simulink model "sim_switc_hover_vol_rotation"  (R2020b)
settings: Solver=VariableStepAuto  StartTime=0.0  StopTime=T  MaxStep=MaxStep  RelTol=RelTol
values from neighbouring files (symbols this model uses):
  a = 400    [switch_hovering_vol_rotation.m]
  b = 500    [switch_hovering_vol_rotation.m]
  controlleur = generateContolleur(drone)    [switch_hovering_vol_rotation.m]
  drone = generateDarko()    [switch_hovering_vol_rotation.m]
  J = 200    [switch_hovering_vol_rotation.m]
  K_complet = [K(:,1:6), [0;0;0;0], K(:,7:12)]    [switch_hovering_vol_rotation.m]
  rule = 1    [switch_hovering_vol_rotation.m]
  S_complet = [S(1:6,1:6), zeros(6,1), S(1:6,7:12); zeros(1,13); S(7:12,1:6), zeros(6,1), S(7:12,7:12)]    [switch_hovering_vol_rotation.m]
  T = 80    [switch_hovering_vol_rotation.m]
  u_eq_hover = drone.G*drone.MASS/(2*drone.Fb(1,1)) * [1;1;0;0]    [switch_hovering_vol_rotation.m]
  x0 = [p_initial; v_initial; q_initial; omega_initial; s]    [switch_hovering_vol_rotation.m]
  x_eq_hover = [[0; 0; 0]; [0; 0; 0]; [1/sqrt(2); 0; -1/sqrt(2);0]; [0; 0; 0]]    [switch_hovering_vol_rotation.m]
undefined symbols (not defined in the file or in its folder): f_initial, q_d_initial, speed
libraries: simulink_extras x5, simulink x3, pid_lib x1, sharedtransform x1
(part 1 of 2)
settings Model: Creator=florian  LastModifiedBy=florian

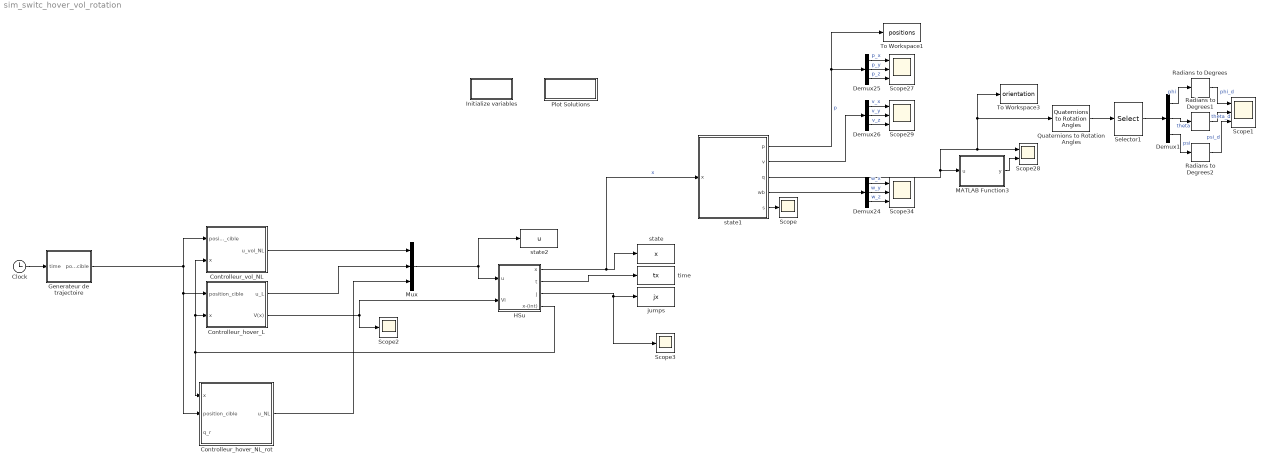
== system sim_switc_hover_vol_rotation ==
  Clock : Clock
  Controlleur_hover_L : Subsystem
  Controlleur_hover_NL_rot : Subsystem
  Controlleur_vol_NL : Subsystem
  Demux{1,24..26} (4 alike) : Demux  Outputs=3
  Generateur de trajectoire : MATLAB Function  TreatAsAtomicUnit=on
  HSu : Subsystem  LoadFcn=set_param(gcb,'LinkStatus','none')
      settings: CopyFcn=|
      | set_param(gcb,'LinkStatus','none'),
      | set_param(gcs, 'MaxStep', 'MaxStep', 'RelTol', 'RelTol','Stop time', 'T')
      mask Display:
      | image(imread('Hcal.jpg'))
      | %plot([5 20 20 5 5],[5 5 20 20 5])
      | %text(8,13,'HyEq_mdl')
      | port_label('output', 1, 'x')
      | port_label('output', 2, 't')
      | port_label('output', 3, 'j')
      | port_label('output', 4, 'x-(int)')
      | port_label('input', 1, 'u')
      | port_label('input', 2, 'V(x)')
  Initialize variables : Subsystem  Priority=-10
      settings: OpenFcn=initialization_di
      mask Display: disp('Double Click\n to Initialize')
  MATLAB Function3 : MATLAB Function  TreatAsAtomicUnit=on
  Mux : Mux  Inputs=3
  Plot Solutions : Subsystem
      settings: OpenFcn=postprocessing_di
      mask Display: disp('Double Click to\n Plot Solutions')
  Quaternions to Rotation Angles : sharedtransform/Quaternions to Rotation Angles  rotationOrder=ZXY  aMode=aMode
      settings: SourceProductBaseCode=AE,PW,MT,UV,VE,VP
  Radians to Degrees : simulink_extras/Transformations/Radians to Degrees
  Radians to Degrees1 : simulink_extras/Transformations/Radians to Degrees
  Radians to Degrees2 : simulink_extras/Transformations/Radians to Degrees
  Scope : Scope
  Scope{1,27,29,34} (4 alike) : Scope  NumInputPorts=3
  Scope2 : Scope
  Scope28 : Scope  NumInputPorts=2
  Scope3 : Scope
  Selector1 : Selector  InputPortWidth=3  IndexOptions=Index vector (dialog)  Indices=[2 3 1]  OutputSizes=1
  To Workspace1 : ToWorkspace  VariableName=positions  SampleTime=-1
  To Workspace3 : ToWorkspace  VariableName=orientation  SampleTime=-1
  jumps : ToWorkspace  VariableName=jx  SampleTime=-1
  state : ToWorkspace  VariableName=x  SampleTime=-1
  state1 : MATLAB Function  TreatAsAtomicUnit=on
  state2 : ToWorkspace  VariableName=u  SampleTime=-1
  time : ToWorkspace  VariableName=tx  SampleTime=-1
  wires:
  Mux/1 -> HSu/1(u), state2/1
  HSu/1(x) -> state1/1(x), state/1  "x"
  HSu/2(t) -> time/1
  HSu/3(j) -> jumps/1, Scope3/1
  Controlleur_hover_L/1(u_L) -> Mux/2
  Generateur de trajectoire/1(position_cible) -> Controlleur_vol_NL/1(position_cible), Controlleur_hover_NL_rot/2(position_cible), Controlleur_hover_L/1(position_cible)
  Controlleur_hover_L/2(V(x)) -> Scope2/1, HSu/2(Vi)
  HSu/4(x-(int)) -> Controlleur_hover_NL_rot/1(x), Controlleur_vol_NL/2(x), Controlleur_hover_L/2(x)
  Demux1/2 -> Radians to Degrees1/1  "theta"
  Quaternions to Rotation Angles/1 -> Selector1/1
  Demux1/3 -> Radians to Degrees2/1  "psi"
  Demux24/2 -> Scope34/2  "w_y"
  Demux26/3 -> Scope29/3  "v_z"
  state1/1(p) -> To Workspace1/1, Demux25/1  "p"
  Demux25/3 -> Scope27/3  "p_z"
  Demux1/1 -> Radians to Degrees/1  "phi"
  Demux25/1 -> Scope27/1  "p_x"
  state1/3(q) -> Scope28/1, To Workspace3/1, Quaternions to Rotation Angles/1, MATLAB Function3/1(u)
  Selector1/1 -> Demux1/1
  Radians to Degrees/1 -> Scope1/1  "phi_d"
  Radians to Degrees1/1 -> Scope1/2  "theta_d"
  Radians to Degrees2/1 -> Scope1/3  "psi_d"
  MATLAB Function3/1(y) -> Scope28/2
  state1/2(v) -> Demux26/1
  Demux26/2 -> Scope29/2  "v_y"
  Demux24/3 -> Scope34/3  "w_z"
  state1/4(wb) -> Demux24/1
  Demux24/1 -> Scope34/1  "w_x"
  Demux26/1 -> Scope29/1  "v_x"
  Demux25/2 -> Scope27/2  "p_y"
  state1/5(s) -> Scope/1
  Controlleur_vol_NL/1(u_vol_NL) -> Mux/1
  Controlleur_hover_NL_rot/1(u_NL) -> Mux/3
  Clock/1 -> Generateur de trajectoire/1(time)

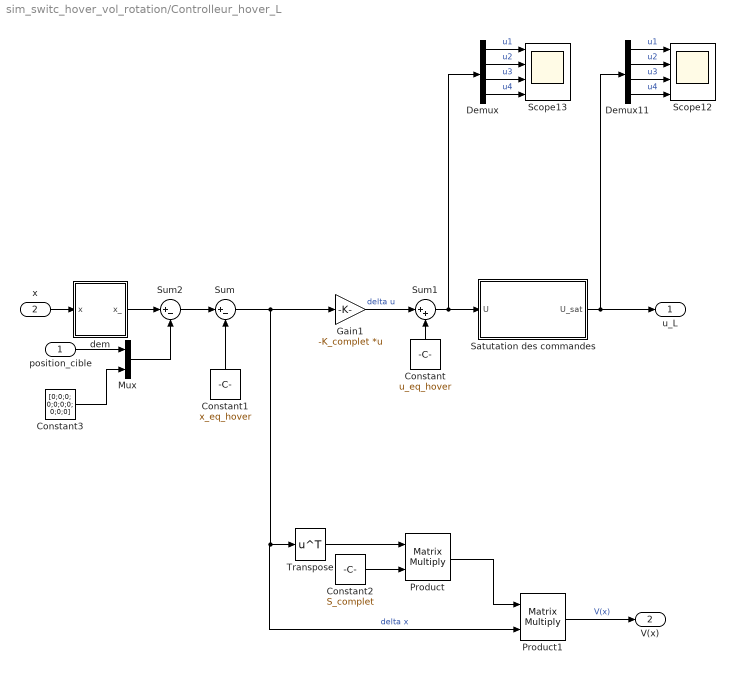
== system sim_switc_hover_vol_rotation/Controlleur_hover_L ==
  position_cible : Inport
  x : Inport  Port=2
  Constant : Constant  Value=u_eq_hover
  Constant1 : Constant  Value=x_eq_hover
  Constant2 : Constant  Value=S_complet
  Constant3 : Constant  Value=[0;0;0; 0;0;0;0; 0;0;0]
  Demux : Demux
  Demux11 : Demux
  Gain1 : Gain  Gain=-K_complet  Multiplication=Matrix(K*u) (u vector)
  Mux : Mux  Inputs=2
  Product : Product  Multiplication=Matrix(*)
  Product1 : Product  Multiplication=Matrix(*)
  Satutation des commandes : Subsystem
  Scope12 : Scope  NumInputPorts=4
  Scope13 : Scope  NumInputPorts=4
  Sum : Sum  Inputs=|+-
  Sum1 : Sum  Inputs=|++
  Sum2 : Sum  Inputs=|+-
  Transpose : Math  Operator=transpose  SaturateOnIntegerOverflow=on
  dem : MATLAB Function  TreatAsAtomicUnit=on
  u_L : Outport
  V(x) : Outport  Port=2
  wires:
  Demux/1 -> Scope13/1  "u1"
  Demux/3 -> Scope13/3  "u3"
  Gain1/1 -> Sum1/1  "delta u"
  Sum1/1 -> Satutation des commandes/1(U), Demux/1
  Sum/1 -> Gain1/1, Product1/2, Transpose/1  "delta x"
  Demux11/3 -> Scope12/3  "u3"
  Satutation des commandes/1(U_sat) -> u_L/1, Demux11/1
  Demux11/2 -> Scope12/2  "u2"
  Product1/1 -> V(x)/1  "V(x)"
  Demux/4 -> Scope13/4  "u4"
  Constant1/1 -> Sum/2
  Transpose/1 -> Product/1
  Product/1 -> Product1/1
  Constant/1 -> Sum1/2
  Demux11/4 -> Scope12/4  "u4"
  Demux/2 -> Scope13/2  "u2"
  Constant2/1 -> Product/2
  Sum2/1 -> Sum/1
  Demux11/1 -> Scope12/1  "u1"
  Mux/1 -> Sum2/2
  position_cible/1 -> Mux/1
  Constant3/1 -> Mux/2
  x/1 -> dem/1(x)
  dem/1(x_) -> Sum2/1

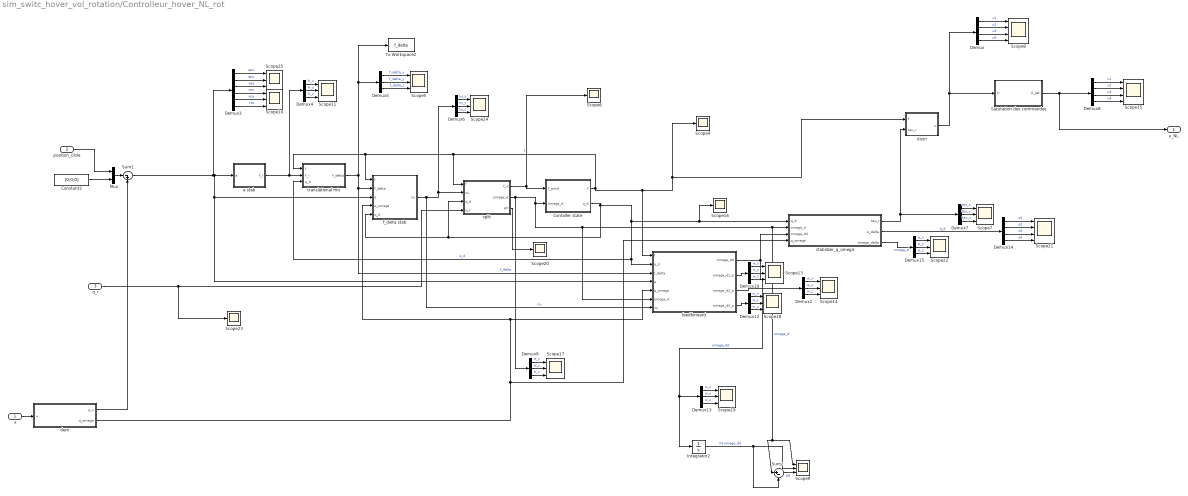
== system sim_switc_hover_vol_rotation/Controlleur_hover_NL_rot ==
  x : Inport
  position_cible : Inport  Port=2
  q_r : Inport  Port=3
  Constant2 : Constant  Value=[0;0;0]
  Contoller state : Subsystem
  Demux : Demux
  Demux{2,4..7,9..10,12..13,15} (10 alike) : Demux  Outputs=3
  Demux14 : Demux
  Demux3 : Demux  Outputs=6
  Demux8 : Demux
  Integrator2 : Integrator
  Mux : Mux  Inputs=2
  Satutation des commandes : Subsystem
  Scope{5,7,9..11,13..14,17..19,22,24..25} (13 alike) : Scope  NumInputPorts=3
  Scope15 : Scope  NumInputPorts=4
  Scope{4,6,16,20,23} (5 alike) : Scope
  Scope21 : Scope  NumInputPorts=4
  Scope8 : Scope  NumInputPorts=4
  Sum1 : Sum  Inputs=|-+
  Sum2 : Sum  Inputs=|+-
  To Workspace2 : ToWorkspace  VariableName=f_delta  SampleTime=-1
  dem : MATLAB Function  TreatAsAtomicUnit=on
  distri : MATLAB Function  TreatAsAtomicUnit=on
  e stab : MATLAB Function  TreatAsAtomicUnit=on
  f_delta stab : MATLAB Function  TreatAsAtomicUnit=on
  feedforward : MATLAB Function  TreatAsAtomicUnit=on
  split : MATLAB Function  TreatAsAtomicUnit=on
  stabilizer_q_omega : MATLAB Function  TreatAsAtomicUnit=on
  translational mis : MATLAB Function  TreatAsAtomicUnit=on
  u_NL : Outport
  wires:
  Demux3/3 -> Scope25/3  "epz"
  Demux15/2 -> Scope22/2  "w_y"
  feedforward/1(omega_dd) -> stabilizer_q_omega/3(omega_dd), Demux13/1, Integrator2/1  "omega_dd"
  split/2(omega_d) -> Demux9/1, feedforward/6(omega_d), Sum2/1, Scope9/1, stabilizer_q_omega/2(omega_d), Contoller state/2(omega_d)  "omega_d"
  Demux3/2 -> Scope25/2  "epy"
  Demux8/4 -> Scope15/4  "u4"
  Demux6/1 -> Scope24/1  "nu_x"
  translational mis/1(f_delta) -> Demux5/1, To Workspace2/1, feedforward/3(f_delta), f_delta stab/2(f_delta)  "f_delta"
  Demux7/2 -> Scope7/2  "tau_y"
  feedforward/3(omega_d2_p) -> Demux2/1
  Demux3/1 -> Scope25/1  "epx"
  Demux8/3 -> Scope15/3  "u3"
  Constant2/1 -> Mux/2
  Demux7/3 -> Scope7/3  "tau_z"
  Demux/3 -> Scope8/3  "u3"
  Demux10/1 -> Scope13/1  "w_x"
  position_cible/1 -> Mux/1
  Demux7/1 -> Scope7/1  "tau_x"
  Satutation des commandes/1(U_sat) -> u_NL/1, Demux8/1
  Demux13/2 -> Scope19/2  "w_y"
  Sum1/1 -> Demux3/1, feedforward/4(e), f_delta stab/3(e), e stab/1(e)
  Demux4/1 -> Scope11/1  "fr_x"
  Demux5/3 -> Scope5/3  "f_delta_z"
  Demux14/1 -> Scope21/1  "q1"
  e stab/1(f_r) -> Demux4/1, translational mis/2(f_r)
  f_delta stab/1(nu) -> feedforward/7(nu), Demux6/1, split/2(nu)  "nu"
  Demux12/2 -> Scope18/2  "w_y"
  q_r/1 -> split/4(q_r), Scope23/1
  Demux6/3 -> Scope24/3  "nu_z"
  Demux8/1 -> Scope15/1  "u1"
  Demux10/2 -> Scope13/2  "w_y"
  Demux9/1 -> Scope17/1  "w_x"
  Mux/1 -> Sum1/1
  Demux12/1 -> Scope18/1  "w_x"
  feedforward/4(omega_d3_p) -> Demux12/1
  Demux/4 -> Scope8/4  "u4"
  Demux8/2 -> Scope15/2  "u2"
  Demux15/1 -> Scope22/1  "w_x"
  Demux5/2 -> Scope5/2  "f_delta_y"
  Demux10/3 -> Scope13/3  "w_z"
  Integrator2/1 -> Sum2/2, Scope9/2  "int omega_dd"
  Demux15/3 -> Scope22/3  "w_z"
  Demux9/2 -> Scope17/2  "w_y"
  Demux2/2 -> Scope14/2  "w_y"
  Demux2/3 -> Scope14/3  "w_z"
  dem/2(q_omega) -> stabilizer_q_omega/4(q_omega), feedforward/5(q_omega), f_delta stab/4(q_omega)
  Demux12/3 -> Scope18/3  "w_z"
  Contoller state/1(f) -> f_delta stab/1(f), translational mis/1(f), split/1(f), feedforward/1(f), Scope4/1, distri/1(f)  "f"
  Demux6/2 -> Scope24/2  "nu_y"
  split/1(f_d) -> Scope6/1, Contoller state/1(f_point)
  Demux/2 -> Scope8/2  "u2"
  Demux13/3 -> Scope19/3  "w_z"
  Demux9/3 -> Scope17/3  "w_z"
  Demux3/4 -> Scope10/1  "vpx"
  Demux2/1 -> Scope14/1  "w_x"
  Demux4/3 -> Scope11/3  "fr_z"
  Contoller state/2(q_d) -> f_delta stab/5(q_d), split/3(q_d), feedforward/2(q_d), translational mis/3(q_d), Scope16/1, stabilizer_q_omega/1(q_d)  "q_d"
  Demux13/1 -> Scope19/1  "w_x"
  Demux3/5 -> Scope10/2  "vpy"
  Demux5/1 -> Scope5/1  "f_delta_x"
  Demux3/6 -> Scope10/3  "vpz"
  Sum2/1 -> Scope9/3  "dif"
  Demux14/2 -> Scope21/2  "q2"
  dem/1(p_v) -> Sum1/2
  Demux4/2 -> Scope11/2  "fr_y"
  stabilizer_q_omega/2(q_delta) -> Demux14/1  "q_d"
  split/3(err) -> Scope20/1
  Demux14/4 -> Scope21/4  "q4"
  Demux/1 -> Scope8/1  "u1"
  stabilizer_q_omega/1(tau_r) -> distri/2(tau_r), Demux7/1
  feedforward/2(omega_d1_p) -> Demux10/1
  stabilizer_q_omega/3(omega_delta) -> Demux15/1  "omega_d"
  distri/1(u) -> Satutation des commandes/1(U), Demux/1
  Demux14/3 -> Scope21/3  "q3"
  x/1 -> dem/1(x)

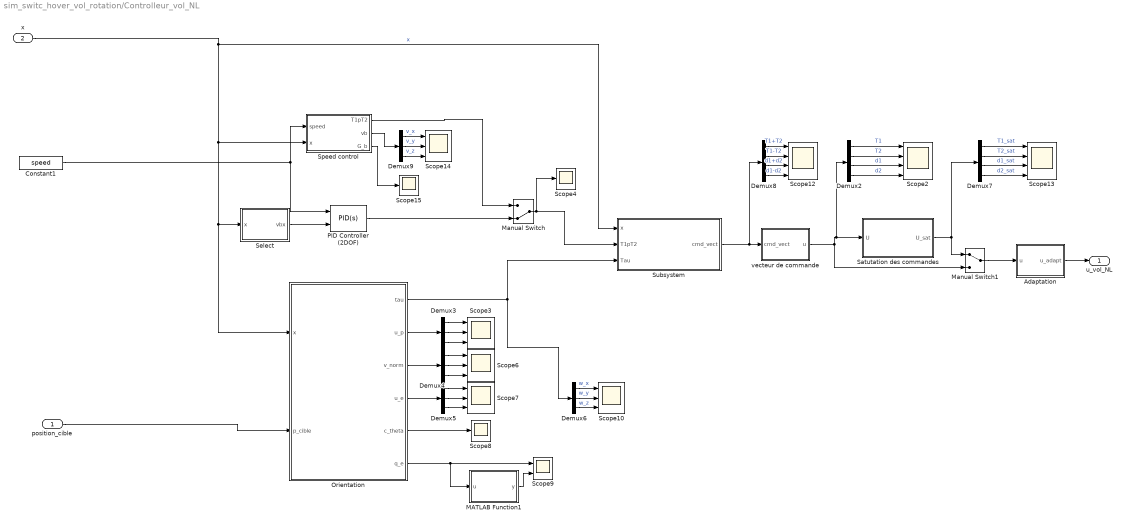
== system sim_switc_hover_vol_rotation/Controlleur_vol_NL ==
  position_cible : Inport
  x : Inport  Port=2
  Adaptation : MATLAB Function  TreatAsAtomicUnit=on
  Constant1 : Constant  Value=speed
  Demux2 : Demux
  Demux{3..6,9} (5 alike) : Demux  Outputs=3
  Demux7 : Demux
  Demux8 : Demux
  MATLAB Function1 : MATLAB Function  TreatAsAtomicUnit=on
  Manual Switch : ManualSwitch  CurrentSetting=0
  Manual Switch1 : ManualSwitch
  Orientation : MATLAB Function  TreatAsAtomicUnit=on
  PID Controller (2DOF) : pid_lib/PID Controller (2DOF)  Controller=PID  Form=Parallel  TimeDomain=Continuous-time  UseExternalTs=off  SampleTime=-1  IntegratorMethod=Forward Euler  FilterMethod=Forward Euler  ControllerParametersSource=internal  P=1  I=1  D=0.1  UseFilter=on  N=100  b=1  c=1  TunerSelectOption=Transfer Function Based (PID Tuner App)  InitialConditionSource=internal  InitialConditionForIntegrator=0  InitialConditionForFilter=0  DifferentiatorICPrevScaledInput=0  ExternalReset=none  TrackingMode=off  Kt=1  LimitOutput=off  SatLimitsSource=internal  UpperSaturationLimit=inf  LowerSaturationLimit=-inf  LinearizeAsGain=on  AntiWindupMode=none  Kb=1  POutMin=[]  POutMax=[]  IOutMin=[]  IOutMax=[]  DOutMin=[]  DOutMax=[]  NOutMin=[]  NOutMax=[]  bOutMin=[]  bOutMax=[]  cOutMin=[]  cOutMax=[]  SumOutMin=[]  SumOutMax=[]  SaturationOutMin=[]  SaturationOutMax=[]  PParamMin=[]  PParamMax=[]  IParamMin=[]  IParamMax=[]  DParamMin=[]  DParamMax=[]  NParamMin=[]  NParamMax=[]  bParamMin=[]  bParamMax=[]  cParamMin=[]  cParamMax=[]  KbParamMin=[]  KbParamMax=[]  KtParamMin=[]  KtParamMax=[]  KbOutMin=[]  KbOutMax=[]  KtOutMin=[]  KtOutMax=[]  IntegratorOutMin=[]  IntegratorOutMax=[]  FilterOutMin=[]  FilterOutMax=[]  SumI1OutMin=[]  SumI1OutMax=[]  SumI2OutMin=[]  SumI2OutMax=[]  SumI3OutMin=[]  SumI3OutMax=[]  SumI4OutMin=[]  SumI4OutMax=[]  SumDOutMin=[]  SumDOutMax=[]  Sum1OutMin=[]  Sum1OutMax=[]  Sum2OutMin=[]  Sum2OutMax=[]  Sum3OutMin=[]  Sum3OutMax=[]  DifferentiatorOutMin=[]  DifferentiatorOutMax=[]  FilterDiffOutCoefMin=[]  FilterDiffOutCoefMax=[]  ReciprocalOutMin=[]  ReciprocalOutMax=[]  SumDenOutMin=[]  SumDenOutMax=[]  SumNumOutMin=[]  SumNumOutMax=[]  DivideOutMin=[]  DivideOutMax=[]  UdiffTsProdOutMin=[]  UdiffTsProdOutMax=[]  NTsProdOutMin=[]  NTsProdOutMax=[]  UintegralTsProdOutMin=[]  UintegralTsProdOutMax=[]  UngainTsProdOutMin=[]  UngainTsProdOutMax=[]  IntegratorContinuousStateAttributes=''  IntegratorStateMustResolveToSignalObject=off  IntegratorRTWStateStorageClass=Auto  FilterContinuousStateAttributes=''  FilterStateMustResolveToSignalObject=off  FilterRTWStateStorageClass=Auto  ParallelPVariant=InternalParameters  IdealPVariant=Disabled  IVariant=InternalParameters  DVariant=InternalParameters  bVariant=InternalParameters  cVariant=InternalParameters  IntegratorVariant=Continuous  SatVariant=Disabled  AWVariant=Passthrough  PCopyVariant=Disabled  TRVariant=Disabled  FdbkBlocksVariant=Forward  IdealPFdbkVariant=Disabled  SatFdbkVariant=Disabled  DerivativeFilterVariant=ContFilter  NVariant=InternalParameters  NCopyVariant=Disabled  FilterICVariant=InternalICsFilter  IntegratorICVariant=InternalICs  ExternalResetVariant=Disabled  TRSumVariant=Passthrough  SumFdbkVariant=Disabled  SumVariant=Sum_PID  TsampFilterVariant=InternalTs  TsampNgainVariant=Passthrough  TsampIntegralVariant=Passthrough  ExternalSaturationOutDataTypeStr=Inherit: Same as second input
      settings: SourceProductBaseCode=SL
  Satutation des commandes : Subsystem
  Scope{3,6..7,10,14} (5 alike) : Scope  NumInputPorts=3
  Scope12 : Scope  NumInputPorts=4
  Scope13 : Scope  NumInputPorts=4
  Scope15 : Scope
  Scope2 : Scope  NumInputPorts=4
  Scope4 : Scope
  Scope8 : Scope
  Scope9 : Scope  NumInputPorts=2
  Select : MATLAB Function  TreatAsAtomicUnit=on
  Speed control : MATLAB Function  TreatAsAtomicUnit=on
  Subsystem : Subsystem
  vecteur de commande : MATLAB Function  TreatAsAtomicUnit=on
  u_vol_NL : Outport
  wires:
  Orientation/4(u_e) -> Demux5/1
  Demux7/1 -> Scope13/1  "T1_sat"
  Demux5/2 -> Scope7/2
  Demux9/3 -> Scope14/3  "v_z"
  Orientation/5(c_theta) -> Scope8/1
  Subsystem/1(cmd_vect) -> Demux8/1, vecteur de commande/1(cmd_vect)
  Demux2/3 -> Scope2/3  "d1"
  Speed control/2(vb) -> Demux9/1
  Orientation/6(q_e) -> MATLAB Function1/1(u), Scope9/1
  Demux6/2 -> Scope10/2  "w_y"
  x/1 -> Subsystem/1(x), Select/1(x), Orientation/1(x), Speed control/2(x)  "x"
  Orientation/3(v_norm) -> Demux4/1
  Orientation/2(u_p) -> Demux3/1
  Demux6/1 -> Scope10/1  "w_x"
  Select/1(vbx) -> PID Controller (2DOF)/2
  Demux6/3 -> Scope10/3  "w_z"
  MATLAB Function1/1(y) -> Scope9/2
  Demux8/3 -> Scope12/3  "d1+d2"
  Orientation/1(tau) -> Subsystem/3(Tau), Demux6/1
  Demux8/4 -> Scope12/4  "d1-d2"
  Demux2/4 -> Scope2/4  "d2"
  Demux4/1 -> Scope6/1
  Demux9/1 -> Scope14/1  "v_x"
  Demux8/2 -> Scope12/2  "T1-T2"
  Demux4/2 -> Scope6/2
  Demux5/3 -> Scope7/3
  Manual Switch/1 -> Scope4/1, Subsystem/2(T1pT2)
  Demux9/2 -> Scope14/2  "v_y"
  Demux7/2 -> Scope13/2  "T2_sat"
  Satutation des commandes/1(U_sat) -> Demux7/1, Manual Switch1/1
  Demux5/1 -> Scope7/1
  Demux3/1 -> Scope3/1
  Speed control/1(T1pT2) -> Manual Switch/1
  Demux2/1 -> Scope2/1  "T1"
  PID Controller (2DOF)/1 -> Manual Switch/2
  Constant1/1 -> Speed control/1(speed), PID Controller (2DOF)/1
  Demux3/3 -> Scope3/3
  Speed control/3(G_b) -> Scope15/1
  Demux8/1 -> Scope12/1  "T1+T2"
  Demux2/2 -> Scope2/2  "T2"
  Demux4/3 -> Scope6/3
  Demux7/3 -> Scope13/3  "d1_sat"
  Demux7/4 -> Scope13/4  "d2_sat"
  vecteur de commande/1(u) -> Demux2/1, Satutation des commandes/1(U), Manual Switch1/2
  Demux3/2 -> Scope3/2
  Manual Switch1/1 -> Adaptation/1(u)
  Adaptation/1(u_adapt) -> u_vol_NL/1
  position_cible/1 -> Orientation/2(p_cible)

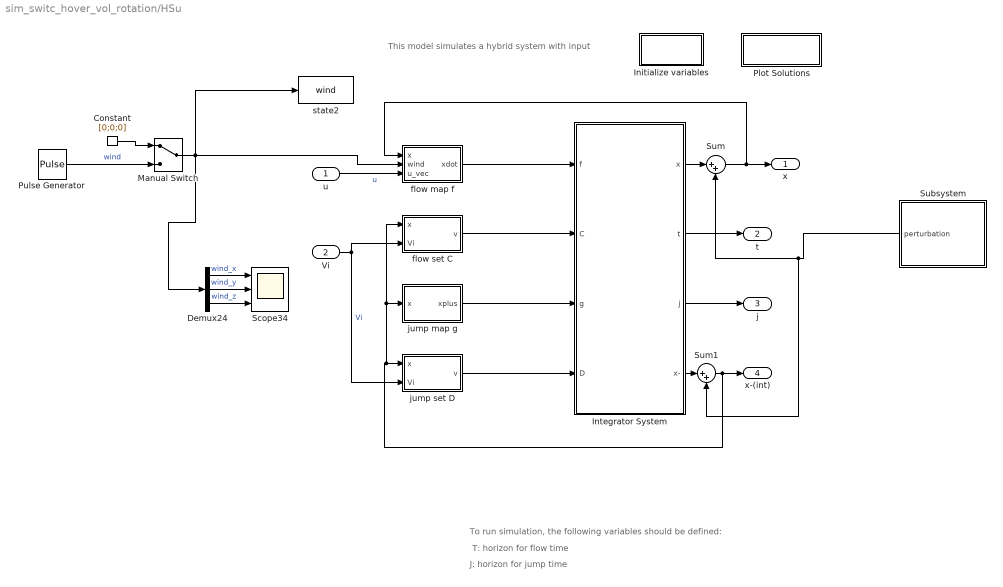
== system sim_switc_hover_vol_rotation/HSu ==
  note: J: horizon for jump time
  note: T: horizon for flow time
  note: To run simulation, the following variables should be defined:
  note: This model simulates a hybrid system with input
  u : Inport
  Vi : Inport  Port=2
  Constant : Constant  Value=[0;0;0]
  Demux24 : Demux  Outputs=3
  Initialize variables : Subsystem  Priority=-10
      settings: OpenFcn=|
      | try
      |      clearvars -except inifile pathfile_in pathfile_pos posfile
      |      cd(pathfile_in);
      |      eval(inifile);
      | catch
      |      [inifile,pathfile_in] = getInitializationfile;
      |      cd(pathfile_in);
      |      inifile = strrep(inifile,'.m','');
      |      eval(inifile);
      | end
      mask Display: disp('Double Click\n to Initialize')
  Integrator System : Subsystem  Priority=2  mask(Hybrid Integrator){T=T, J=J, x0=x0}
      mask prompts: T "Flow Horizon"; J "Jump Horizon"; x0 "Initial Condition"
      mask help:
      | This block integrates the state of the hybrid system defined by the flow map f (first input), the flow set C (second input), the jump map g (third input) and the jump set D (fourth input).
      | Starting from the initial condition x0 (last mask parameter), the system's state x evolves continuously within the set C, according to f(x,u), but is also subject to jumps within D, according to g(x,u).
      | The block also stops the simulation when the time t is greater than the flow horizon T (first mask parameter), or when the number of jumps j is greater than the jump horizon J (second mask parameter).
      | The outputs of the blocks are respectively x(t), t, j, x(t-).
      mask Help:
      | This block integrates the state of the hybrid system defined by the flow map f (first input), the flow set C (second input), the jump map g (third input) and the jump set D (fourth input).
      | <br>
      | Starting from the initial condition x0 (last mask parameter), the system's state x evolves continuously within the set C, according to f(x,u), but is also subject to jumps within D, according to g(x,u).
      | <br>
      | The block also stops the simulation when the time t is greater than the flow horizon T (first mask parameter), or when the number of jumps j is greater than the jump horizon J (second mask parameter).
      | <br>
      | The outputs of the blocks are respectively x(t), t, j, x(t-).
      | <br>
      | You can right click on the block and "Look under mask" to see what's inside the block.
      | Finally, refer to the manual (HybridSimulator_vXX.pdf) for more detailed information on how this hybrid simulator works.
  Manual Switch : ManualSwitch
  Plot Solutions : Subsystem
      settings: OpenFcn=|
      | try
      |      cd(pathfile_pos);
      |      eval(posfile);
      | catch
      |      [posfile,pathfile_pos] = getInitializationfile;
      |      cd(pathfile_pos);
      |      posfile = strrep(posfile,'.m','');
      |      eval(posfile);
      | end
      mask Display: disp('Double Click to\n Plot Solutions')
  Pulse Generator : DiscretePulseGenerator  PulseType=Time based  Amplitude=1.9  Period=10  PulseWidth=30  PhaseDelay=5
  Scope34 : Scope  NumInputPorts=3
  Subsystem : Subsystem
  Sum : Sum  Inputs=|++
  Sum1 : Sum  Inputs=|++
  flow map f : MATLAB Function  TreatAsAtomicUnit=on
  flow set C : MATLAB Function  TreatAsAtomicUnit=on
  jump map g : MATLAB Function  Priority=2  TreatAsAtomicUnit=on
  jump set D : MATLAB Function  TreatAsAtomicUnit=on
  state2 : ToWorkspace  VariableName=wind  SampleTime=-1
  x : Outport
  t : Outport  Port=2
  j : Outport  Port=3
  x-(int) : Outport  Port=4
  wires:
  jump map g/1(xplus) -> Integrator System/3(g)
  jump set D/1(v) -> Integrator System/4(D)
  u/1 -> flow map f/3(u_vec)  "u"
  Integrator System/3(j) -> j/1
  Integrator System/2(t) -> t/1
  flow set C/1(v) -> Integrator System/2(C)
  flow map f/1(xdot) -> Integrator System/1(f)
  Vi/1 -> jump set D/2(Vi), flow set C/2(Vi)  "Vi"
  Constant/1 -> Manual Switch/1
  Manual Switch/1 -> Demux24/1, state2/1, flow map f/2(wind)
  Demux24/1 -> Scope34/1  "wind_x"
  Demux24/2 -> Scope34/2  "wind_y"
  Demux24/3 -> Scope34/3  "wind_z"
  Pulse Generator/1 -> Manual Switch/2  "wind"
  Sum1/1 -> flow set C/1(x), jump map g/1(x), jump set D/1(x), x-(int)/1
  Subsystem/1(perturbation) -> Sum/2, Sum1/2
  Integrator System/1(x) -> Sum/1
  Sum/1 -> flow map f/1(x), x/1
  Integrator System/4(x-) -> Sum1/1

== system sim_switc_hover_vol_rotation/Initialize variables ==

== system sim_switc_hover_vol_rotation/Plot Solutions ==

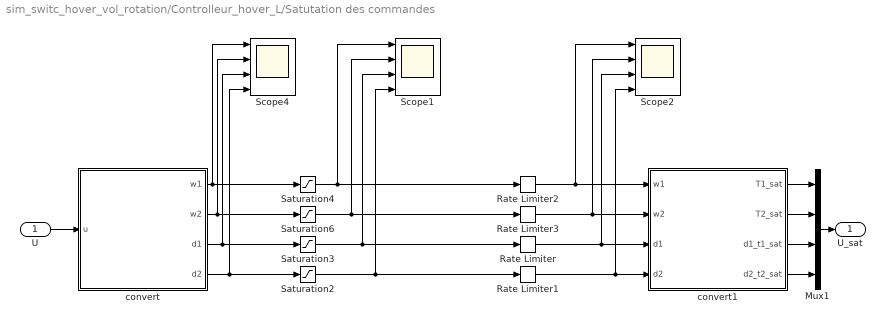
== system sim_switc_hover_vol_rotation/Controlleur_hover_L/Satutation des commandes ==
  U : Inport
  Mux1 : Mux
  Rate Limiter : RateLimiter  RisingSlewLimit=drone.ELEVON_RATE_CHANGE  FallingSlewLimit=-drone.ELEVON_RATE_CHANGE  SampleTimeMode=inherited
  Rate Limiter1 : RateLimiter  RisingSlewLimit=drone.ELEVON_RATE_CHANGE  FallingSlewLimit=-drone.ELEVON_RATE_CHANGE  SampleTimeMode=inherited
  Rate Limiter2 : RateLimiter  RisingSlewLimit=drone.MOTOR_RATE_CHANGE  FallingSlewLimit=-drone.MOTOR_RATE_CHANGE  SampleTimeMode=inherited
  Rate Limiter3 : RateLimiter  RisingSlewLimit=drone.MOTOR_RATE_CHANGE  FallingSlewLimit=-drone.MOTOR_RATE_CHANGE  SampleTimeMode=inherited
  Saturation2 : Saturate  UpperLimit=30*(pi/180)  LowerLimit=-30*(pi/180)
  Saturation3 : Saturate  UpperLimit=30*(pi/180)  LowerLimit=-30*(pi/180)
  Saturation4 : Saturate  UpperLimit=1000  LowerLimit=200
  Saturation6 : Saturate  UpperLimit=1000  LowerLimit=200
  Scope1 : Scope  NumInputPorts=4
  Scope2 : Scope  NumInputPorts=4
  Scope4 : Scope  NumInputPorts=4
  convert : MATLAB Function  TreatAsAtomicUnit=on
  convert1 : MATLAB Function  TreatAsAtomicUnit=on
  U_sat : Outport
  wires:
  convert/1(w1) -> Saturation4/1, Scope4/1
  Saturation3/1 -> Rate Limiter/1, Scope1/3
  convert/2(w2) -> Scope4/2, Saturation6/1
  convert/3(d1) -> Scope4/3, Saturation3/1
  convert/4(d2) -> Saturation2/1, Scope4/4
  convert1/1(T1_sat) -> Mux1/1
  convert1/4(d2_t2_sat) -> Mux1/4
  Mux1/1 -> U_sat/1
  convert1/2(T2_sat) -> Mux1/2
  convert1/3(d1_t1_sat) -> Mux1/3
  Saturation2/1 -> Rate Limiter1/1, Scope1/4
  Rate Limiter/1 -> Scope2/3, convert1/3(d1)
  Saturation6/1 -> Rate Limiter3/1, Scope1/2
  Saturation4/1 -> Rate Limiter2/1, Scope1/1
  Rate Limiter1/1 -> Scope2/4, convert1/4(d2)
  Rate Limiter2/1 -> Scope2/1, convert1/1(w1)
  Rate Limiter3/1 -> Scope2/2, convert1/2(w2)
  U/1 -> convert/1(u)

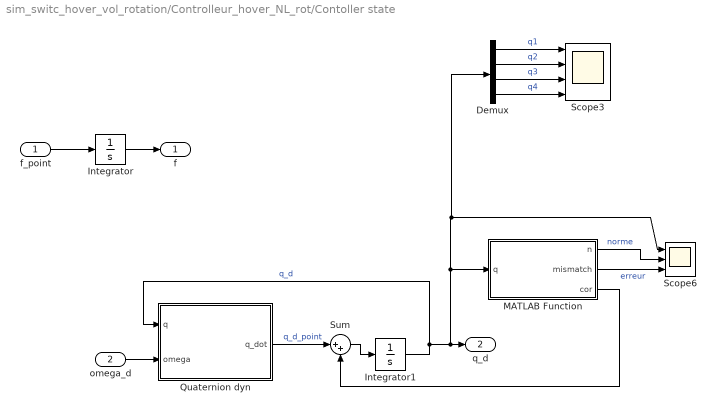
== system sim_switc_hover_vol_rotation/Controlleur_hover_NL_rot/Contoller state ==
  f_point : Inport
  omega_d : Inport  Port=2
  Demux : Demux
  Integrator : Integrator  InitialCondition=f_initial
  Integrator1 : Integrator  InitialCondition=q_d_initial
  MATLAB Function : MATLAB Function  TreatAsAtomicUnit=on
  Quaternion dyn : MATLAB Function  TreatAsAtomicUnit=on
  Scope3 : Scope  NumInputPorts=4
  Scope6 : Scope  NumInputPorts=3
  Sum : Sum  Inputs=|++
  f : Outport
  q_d : Outport  Port=2
  wires:
  Integrator/1 -> f/1
  f_point/1 -> Integrator/1
  Integrator1/1 -> Quaternion dyn/1(q), Demux/1, Scope6/1, MATLAB Function/1(q), q_d/1  "q_d"
  omega_d/1 -> Quaternion dyn/2(omega)
  Quaternion dyn/1(q_dot) -> Sum/1  "q_d_point"
  Sum/1 -> Integrator1/1
  MATLAB Function/3(cor) -> Sum/2
  MATLAB Function/1(n) -> Scope6/2  "norme"
  MATLAB Function/2(mismatch) -> Scope6/3  "erreur"
  Demux/3 -> Scope3/3  "q3"
  Demux/2 -> Scope3/2  "q2"
  Demux/1 -> Scope3/1  "q1"
  Demux/4 -> Scope3/4  "q4"

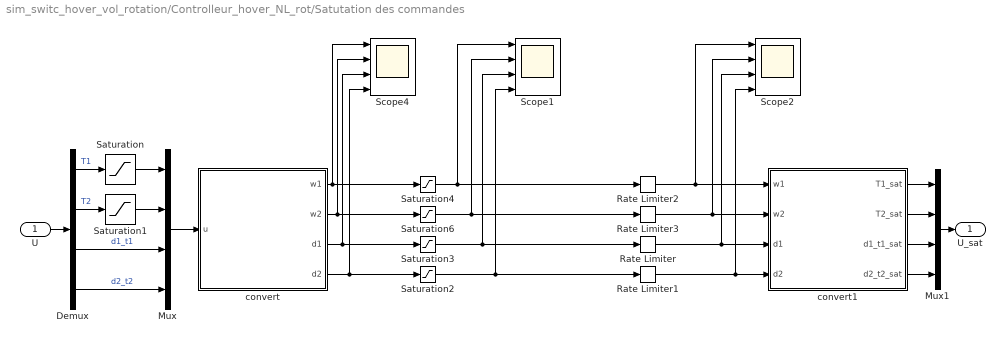
== system sim_switc_hover_vol_rotation/Controlleur_hover_NL_rot/Satutation des commandes ==
  U : Inport
  Demux : Demux
  Mux : Mux
  Mux1 : Mux
  Rate Limiter : RateLimiter  RisingSlewLimit=drone.ELEVON_RATE_CHANGE  FallingSlewLimit=-drone.ELEVON_RATE_CHANGE  SampleTimeMode=inherited
  Rate Limiter1 : RateLimiter  RisingSlewLimit=drone.ELEVON_RATE_CHANGE  FallingSlewLimit=-drone.ELEVON_RATE_CHANGE  SampleTimeMode=inherited
  Rate Limiter2 : RateLimiter  RisingSlewLimit=drone.MOTOR_RATE_CHANGE  FallingSlewLimit=-drone.MOTOR_RATE_CHANGE  SampleTimeMode=inherited
  Rate Limiter3 : RateLimiter  RisingSlewLimit=drone.MOTOR_RATE_CHANGE  FallingSlewLimit=-drone.MOTOR_RATE_CHANGE  SampleTimeMode=inherited
  Saturation : Saturate  UpperLimit=100  LowerLimit=0.001
  Saturation1 : Saturate  UpperLimit=100  LowerLimit=0.001
  Saturation2 : Saturate  UpperLimit=30*(pi/180)  LowerLimit=-30*(pi/180)
  Saturation3 : Saturate  UpperLimit=30*(pi/180)  LowerLimit=-30*(pi/180)
  Saturation4 : Saturate  UpperLimit=1000  LowerLimit=200
  Saturation6 : Saturate  UpperLimit=1000  LowerLimit=200
  Scope1 : Scope  NumInputPorts=4
  Scope2 : Scope  NumInputPorts=4
  Scope4 : Scope  NumInputPorts=4
  convert : MATLAB Function  TreatAsAtomicUnit=on
  convert1 : MATLAB Function  TreatAsAtomicUnit=on
  U_sat : Outport
  wires:
  U/1 -> Demux/1
  Demux/4 -> Mux/4  "d2_t2"
  Demux/1 -> Saturation/1  "T1"
  Demux/3 -> Mux/3  "d1_t1"
  Demux/2 -> Saturation1/1  "T2"
  Saturation/1 -> Mux/1
  Mux/1 -> convert/1(u)
  convert/1(w1) -> Saturation4/1, Scope4/1
  Saturation3/1 -> Rate Limiter/1, Scope1/3
  convert/2(w2) -> Scope4/2, Saturation6/1
  convert/3(d1) -> Scope4/3, Saturation3/1
  convert/4(d2) -> Saturation2/1, Scope4/4
  convert1/1(T1_sat) -> Mux1/1
  convert1/4(d2_t2_sat) -> Mux1/4
  Mux1/1 -> U_sat/1
  Saturation1/1 -> Mux/2
  convert1/2(T2_sat) -> Mux1/2
  convert1/3(d1_t1_sat) -> Mux1/3
  Saturation2/1 -> Rate Limiter1/1, Scope1/4
  Rate Limiter/1 -> Scope2/3, convert1/3(d1)
  Saturation6/1 -> Rate Limiter3/1, Scope1/2
  Saturation4/1 -> Rate Limiter2/1, Scope1/1
  Rate Limiter1/1 -> Scope2/4, convert1/4(d2)
  Rate Limiter2/1 -> Scope2/1, convert1/1(w1)
  Rate Limiter3/1 -> Scope2/2, convert1/2(w2)

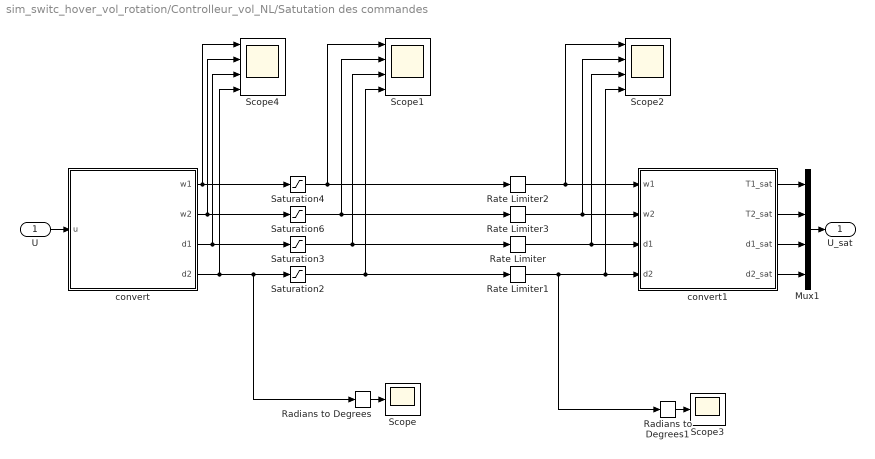
== system sim_switc_hover_vol_rotation/Controlleur_vol_NL/Satutation des commandes ==
  U : Inport
  Mux1 : Mux
  Radians to Degrees : simulink_extras/Transformations/Radians to Degrees
  Radians to Degrees1 : simulink_extras/Transformations/Radians to Degrees
  Rate Limiter : RateLimiter  RisingSlewLimit=drone.ELEVON_RATE_CHANGE  FallingSlewLimit=-drone.ELEVON_RATE_CHANGE  SampleTimeMode=inherited
  Rate Limiter1 : RateLimiter  RisingSlewLimit=drone.ELEVON_RATE_CHANGE  FallingSlewLimit=-drone.ELEVON_RATE_CHANGE  SampleTimeMode=inherited
  Rate Limiter2 : RateLimiter  RisingSlewLimit=drone.MOTOR_RATE_CHANGE  FallingSlewLimit=-drone.MOTOR_RATE_CHANGE  SampleTimeMode=inherited
  Rate Limiter3 : RateLimiter  RisingSlewLimit=drone.MOTOR_RATE_CHANGE  FallingSlewLimit=-drone.MOTOR_RATE_CHANGE  SampleTimeMode=inherited
  Saturation2 : Saturate  UpperLimit=30*(pi/180)  LowerLimit=-30*(pi/180)
  Saturation3 : Saturate  UpperLimit=30*(pi/180)  LowerLimit=-30*(pi/180)
  Saturation4 : Saturate  UpperLimit=1000  LowerLimit=200
  Saturation6 : Saturate  UpperLimit=1000  LowerLimit=200
  Scope : Scope
  Scope1 : Scope  NumInputPorts=4
  Scope2 : Scope  NumInputPorts=4
  Scope3 : Scope
  Scope4 : Scope  NumInputPorts=4
  convert : MATLAB Function  TreatAsAtomicUnit=on
  convert1 : MATLAB Function  TreatAsAtomicUnit=on
  U_sat : Outport
  wires:
  convert/1(w1) -> Saturation4/1, Scope4/1
  convert/2(w2) -> Scope4/2, Saturation6/1
  convert/3(d1) -> Scope4/3, Saturation3/1
  convert1/1(T1_sat) -> Mux1/1
  convert1/4(d2_sat) -> Mux1/4
  Mux1/1 -> U_sat/1
  convert1/2(T2_sat) -> Mux1/2
  convert1/3(d1_sat) -> Mux1/3
  Rate Limiter/1 -> Scope2/3, convert1/3(d1)
  Saturation6/1 -> Rate Limiter3/1, Scope1/2
  Saturation4/1 -> Rate Limiter2/1, Scope1/1
  Rate Limiter2/1 -> Scope2/1, convert1/1(w1)
  Rate Limiter3/1 -> Scope2/2, convert1/2(w2)
  U/1 -> convert/1(u)
  Saturation3/1 -> Rate Limiter/1, Scope1/3
  Saturation2/1 -> Rate Limiter1/1, Scope1/4
  convert/4(d2) -> Radians to Degrees/1, Saturation2/1, Scope4/4
  Radians to Degrees/1 -> Scope/1
  Radians to Degrees1/1 -> Scope3/1
  Rate Limiter1/1 -> Radians to Degrees1/1, Scope2/4, convert1/4(d2)

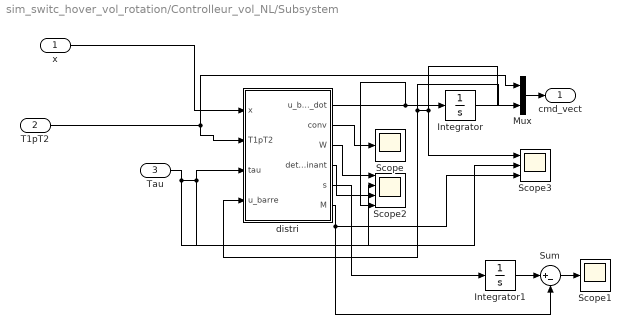
== system sim_switc_hover_vol_rotation/Controlleur_vol_NL/Subsystem ==
  x : Inport
  T1pT2 : Inport  Port=2
  Tau : Inport  Port=3
  Integrator : Integrator  InitialCondition=[0;0;0]
  Integrator1 : Integrator
  Mux : Mux  Inputs=2
  Scope : Scope
  Scope1 : Scope
  Scope2 : Scope  NumInputPorts=4
  Scope3 : Scope  NumInputPorts=3
  Sum : Sum  Inputs=|+-
  distri : MATLAB Function  TreatAsAtomicUnit=on
  cmd_vect : Outport
  wires:
  Integrator/1 -> distri/4(u_barre), Scope3/1, Mux/2
  Mux/1 -> cmd_vect/1
  distri/2(conv) -> Scope/1
  distri/4(determinant) -> Scope2/3
  distri/3(W) -> Scope2/1
  distri/5(s) -> Integrator1/1
  Integrator1/1 -> Sum/1
  distri/6(M) -> Sum/2, Scope3/3
  Sum/1 -> Scope1/1
  x/1 -> distri/1(x)
  T1pT2/1 -> distri/2(T1pT2), Mux/1
  Tau/1 -> Scope3/2, Scope2/2, distri/3(tau)
  distri/1(u_barre_dot) -> Scope2/4, Integrator/1

== system sim_switc_hover_vol_rotation/HSu/Initialize variables ==

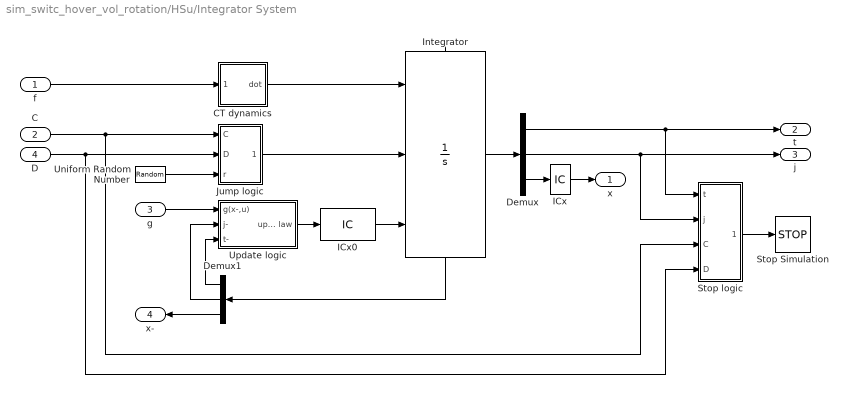
== system sim_switc_hover_vol_rotation/HSu/Integrator System ==
  f : Inport
  C : Inport  Port=2
  g : Inport  Port=3
  D : Inport  Port=4
  CT dynamics : Subsystem
  Demux : Demux  Outputs=[1 1 -1]
  Demux1 : Demux  Outputs=[1 1 -1]
  ICx : InitialCondition  Value=x0
  ICx0 : InitialCondition  Value=[0; 0; x0(:)]
  Integrator : Integrator  ExternalReset=level hold  InitialConditionSource=external  ShowStatePort=on  ZeroCross=off
  Jump logic : Subsystem
  Stop Simulation : Stop
  Stop logic : Subsystem
  Uniform Random Number : UniformRandomNumber  Minimum=0  Seed=abs(floor(100*rand))  SampleTime=0
  Update logic : Subsystem
  x : Outport
  t : Outport  Port=2
  j : Outport  Port=3
  x- : Outport  Port=4
  wires:
  ICx0/1 -> Integrator/3
  ICx/1 -> x/1
  Demux/3 -> ICx/1
  Integrator/State -> Demux1/1
  Demux/2 -> j/1, Stop logic/2(j)
  Demux/1 -> t/1, Stop logic/1(t)
  Update logic/1(update law) -> ICx0/1
  CT dynamics/1(dot) -> Integrator/1
  Stop logic/1(stop) -> Stop Simulation/1
  Integrator/1 -> Demux/1
  C/1 -> Stop logic/3(C), Jump logic/1(C)
  D/1 -> Stop logic/4(D), Jump logic/2(D)
  f/1 -> CT dynamics/1(f(x,u))
  Demux1/3 -> x-/1
  Jump logic/1(jump) -> Integrator/2
  Uniform Random Number/1 -> Jump logic/3(r)
  g/1 -> Update logic/1(g(x-,u))
  Demux1/1 -> Update logic/3(t-)
  Demux1/2 -> Update logic/2(j-)

== system sim_switc_hover_vol_rotation/HSu/Plot Solutions ==

== system sim_switc_hover_vol_rotation/HSu/Subsystem ==
  Clock : Clock
  MATLAB Function : MATLAB Function  TreatAsAtomicUnit=on
  perturbation : Outport
  wires:
  Clock/1 -> MATLAB Function/1(t)
  MATLAB Function/1(y) -> perturbation/1

== system sim_switc_hover_vol_rotation/HSu/Integrator System/CT dynamics ==
  f(x,u) : Inport
  Flows : Constant
  Jumps : Constant  Value=0
  Mux : Mux  Inputs=[1 1 -1]
  dot : Outport
  wires:
  Jumps/1 -> Mux/2
  Flows/1 -> Mux/1
  Mux/1 -> dot/1
  f(x,u)/1 -> Mux/3

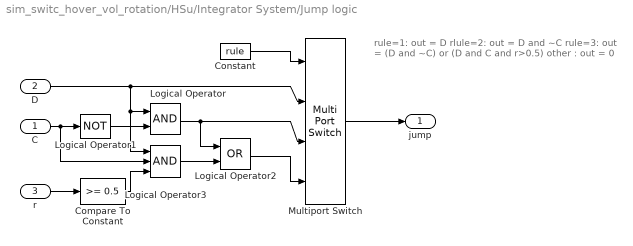
== system sim_switc_hover_vol_rotation/HSu/Integrator System/Jump logic ==
  note: rule=1:  out = D
      | rlule=2: out = D and ~C
      | rule=3:  out = (D and ~C)  or (D and C and r>0.5)
      | other :  out = 0
  C : Inport
  D : Inport  Port=2
  r : Inport  Port=3
  Compare To Constant : simulink/Logic and Bit Operations/Compare To Constant  relop=>=  const=0.5  OutDataTypeStr=uint8
  Constant : Constant  Value=rule
  Logical Operator : Logic  AllPortsSameDT=off  OutDataTypeStr=boolean
  Logical Operator1 : Logic  Operator=NOT  Inputs=1  AllPortsSameDT=off  OutDataTypeStr=boolean
  Logical Operator2 : Logic  Operator=OR  AllPortsSameDT=off  OutDataTypeStr=boolean
  Logical Operator3 : Logic  Inputs=3  AllPortsSameDT=off  OutDataTypeStr=boolean
  Multiport Switch : MultiPortSwitch
  jump : Outport
  wires:
  Constant/1 -> Multiport Switch/1
  D/1 -> Logical Operator3/1, Logical Operator/1, Multiport Switch/2
  r/1 -> Compare To Constant/1
  C/1 -> Logical Operator3/2, Logical Operator1/1
  Logical Operator1/1 -> Logical Operator/2
  Logical Operator/1 -> Multiport Switch/3, Logical Operator2/1
  Logical Operator2/1 -> Multiport Switch/4
  Multiport Switch/1 -> jump/1
  Compare To Constant/1 -> Logical Operator3/3
  Logical Operator3/1 -> Logical Operator2/2

== system sim_switc_hover_vol_rotation/HSu/Integrator System/Stop logic ==
  t : Inport
  j : Inport  Port=2
  C : Inport  Port=3
  D : Inport  Port=4
  "Flow Horizon, T" : simulink/Logic and Bit Operations/Compare To Constant  relop=>=  const=T  OutDataTypeStr=uint8  ZeroCross=off
  "Jump Horizon, J" : simulink/Logic and Bit Operations/Compare To Constant  relop=>=  const=J  OutDataTypeStr=uint8  ZeroCross=off
  Logical Operator : Logic  Operator=NOR  AllPortsSameDT=off  OutDataTypeStr=boolean
  Logical Operator1 : Logic  Operator=OR  Inputs=3  AllPortsSameDT=off  OutDataTypeStr=boolean
  stop : Outport
  wires:
  "Flow Horizon, T"/1 -> Logical Operator1/1
  "Jump Horizon, J"/1 -> Logical Operator1/2
  Logical Operator/1 -> Logical Operator1/3
  D/1 -> Logical Operator/2
  t/1 -> "Flow Horizon, T"/1
  j/1 -> "Jump Horizon, J"/1
  C/1 -> Logical Operator/1
  Logical Operator1/1 -> stop/1

== system sim_switc_hover_vol_rotation/HSu/Integrator System/Update logic ==
  g(x-,u) : Inport
  j- : Inport  Port=2
  t- : Inport  Port=3
  Constant : Constant
  Mux1 : Mux  Inputs=[1 1 -1]
  Sum : Sum  Inputs=|++
  update law : Outport
  wires:
  Sum/1 -> Mux1/2
  Mux1/1 -> update law/1
  j-/1 -> Sum/1
  g(x-,u)/1 -> Mux1/3
  t-/1 -> Mux1/1
  Constant/1 -> Sum/2

== matlab function sim_switc_hover_vol_rotation/Controlleur_hover_NL_rot/feedforward ==
  data: f input; omega_dd output; q_d input; f_delta input; e input; q_omega input; omega_d input; nu input; controlleur parameter; drone parameter; omega_d1_p output; omega_d2_p output; omega_d3_p output
function [omega_dd, omega_d1_p, omega_d2_p, omega_d3_p]  = feedforward(f, q_d, f_delta,e, q_omega,omega_d, nu, controlleur, drone)
%#codegen

d_etoile = controlleur.d_etoile;
kpp = controlleur.kpp;
kpd = controlleur.kpd;
k_delta = controlleur.k_delta;
m = drone.MASS;

ep = e(1:3);
ev = e(4:6);

q = q_omega(1:4);
omega = q_omega(5:7);

R = q2dcm(q);
Rd = q2dcm(q_d);

omega_d1_p = -(1/(f^2)) * skew_sym(d_etoile) * Rd' * nu * ( Rd * d_etoile)' * nu;
omega_d2_p = -(1/(f))* skew_sym(d_etoile) * skew_sym(omega_d) * Rd' * nu;

Gain = (kpd^2/m^2 - kpp/m);

ep_term = - Gain*kpp*ep;
ev_term = (kpp*kpd/m - Gain*kpd)*ev;
f_delta_term = (Gain + (kpd/m + k_delta)*k_delta)*f_delta;
f_term = (Gain*(R-Rd) + kpd/m * (Rd*skew_sym(omega_d) - R*skew_sym(omega)))*d_etoile* f;
nu_term = kpd/m * (Rd-R) * d_etoile * (Rd*d_etoile)'* nu;

omega_d3_p = (1/f) * skew_sym(d_etoile) * Rd'* (ep_term + ev_term + f_delta_term + f_term + nu_term); 

omega_dd = omega_d1_p + omega_d2_p + omega_d3_p ; %

== matlab function sim_switc_hover_vol_rotation/Controlleur_hover_NL_rot/Contoller state/MATLAB Function ==
  data: n output; q input; mismatch output; cor output
function [n, mismatch, cor] = fcn(q)
%#codegen
n = norm(q);
mismatch = 1-norm(q);
cor = mismatch*q;

== matlab function sim_switc_hover_vol_rotation/Controlleur_hover_NL_rot/Satutation des commandes/convert ==
  data: u input; w1 output; drone parameter; w2 output; d1 output; d2 output
function [w1, w2, d1, d2] = convert(u, drone)
%#codegen
kf = drone.PROP_KP;

T1 = u(1);
T2 = u(2);
d1_T1 = u(3);
d2_T2 = u(4);

w1 = sqrt(T1/kf);
w2 = sqrt(T2/kf);
d1 = d1_T1/T1;
d2 = d2_T2/T2;

== matlab function sim_switc_hover_vol_rotation/Controlleur_hover_NL_rot/Contoller state/Quaternion dyn ==
  data: q input; q_dot output; omega input
function q_dot = q_dyn(q, omega)
%#codegen

eta = q(1);
eps = q(2:4);

A = [-eps';  eta*eye(3)+skew_sym(eps)];
q_dot = 1/2*A*omega;

== matlab function sim_switc_hover_vol_rotation/Controlleur_hover_NL_rot/Satutation des commandes/convert1 ==
  data: w1 input; w2 input; d1 input; d2 input; T1_sat output; T2_sat output; drone parameter; d1_t1_sat output; d2_t2_sat output
function [T1_sat, T2_sat, d1_t1_sat, d2_t2_sat] = convert2(w1, w2, d1, d2, drone)
%#codegen
kf = drone.PROP_KP;

T1_sat = kf*w1^2;
d1_t1_sat = d1*T1_sat;
T2_sat = kf*w2^2;
d2_t2_sat = d2*T2_sat;

== matlab function sim_switc_hover_vol_rotation/HSu/flow map f ==
  data: x input; wind input; xdot output; u_vec input; drone parameter
function xdot = f(x, wind, u_vec, drone)
%--------------------------------------------------------------------------
% Matlab M-file Project: HyEQ Toolbox @  Hybrid Systems Laboratory (HSL), 
% https://hybrid.soe.ucsc.edu/software
% http://hybridsimulator.wordpress.com/
%--------------------------------------------------------------------------
% Project: Simulation of a hybrid system
% Description: Flow map
%--------------------------------------------------------------------------
%--------------------------------------------------------------------------
%   See also HYEQSOLVER, PLOTARC, PLOTARC3, PLOTFLOWS, PLOTHARC,
%   PLOTHARCCOLOR, PLOTHARCCOLOR3D, PLOTHYBRIDARC, PLOTJUMPS.
%   Copyright @ Hybrid Systems Laboratory (HSL),
%   Revision: 0.0.0.3 Date: 05/20/2015 3:42:00
%--------------------------------------------------------------------------
% flow map: xdot=f(x,u);

%% physical constants
% gravity
g = drone.G;
% vehicle mass
m = drone.MASS;
% vehicle inertia matrix
J = drone.INERTIA; % [3x3 real symmetric] in body axis

%% state demultiplexing
% p = x(1:3);
v = x(4:6);
q  = x(7:10);
wb = x(11:13);
s = x(14);

%% Commande switch s = 0 => contolleur vol L, s = 1 => contolleur hover L , s = 2 => contolleur hover NL rot

if(s == 0)
    u = u_vec(1:4);
elseif(s == 1)
    u = u_vec(5:8);
elseif(s == 2)
    u = u_vec(9:12);
end
    

Rq = q2dcm(q);

[Fp, Mp] = external_force_moment(x, u, wind, drone);

% position
dpdt = v;

% kinematics
dvdt =  -[0;0;g] + (1/m)*Rq*drone.Fb*u + (1/m)*Rq*Fp; 

%% quaternion derivative
eta = q(1);
eps = q(2:4);

dqdt = (1/2)*[-eps'; eta*eye(3) + skew_sym(eps)]*wb;

%% angular velocity derivative
% kinematics
dwdt = -J\cross(wb, J*wb) + J\(drone.Mb*u) + J\Mp;


%% derivative multiplexing
xdot = [dpdt; dvdt; dqdt; dwdt; 0] ;

== matlab function sim_switc_hover_vol_rotation/HSu/flow set C ==
  data: x input; v output; Vi input; a parameter; b parameter
function v   = C(x, Vi, a, b) 
%--------------------------------------------------------------------------
% Matlab M-file Project: HyEQ Toolbox @  Hybrid Systems Laboratory (HSL), 
% https://hybrid.soe.ucsc.edu/software
% http://hybridsimulator.wordpress.com/
%--------------------------------------------------------------------------
% Project: Simulation of a hybrid system
% Description: Flow set
%--------------------------------------------------------------------------
%--------------------------------------------------------------------------
%   See also HYEQSOLVER, PLOTARC, PLOTARC3, PLOTFLOWS, PLOTHARC,
%   PLOTHARCCOLOR, PLOTHARCCOLOR3D, PLOTHYBRIDARC, PLOTJUMPS.
%   Copyright @ Hybrid Systems Laboratory (HSL),
%   Revision: 0.0.0.3 Date: 05/20/2015 3:42:00
%
%state
s = x(14);


if (((Vi <= b ) && (s == 0)) || ((Vi >= a ) && (s == 1)))  % flow condition
    v = 1;  % report flow
else
    v = 0;   % do not report flow
end

== matlab function sim_switc_hover_vol_rotation/HSu/jump map g ==
  data: x input; xplus output
function xplus = g(x)
%--------------------------------------------------------------------------
% Matlab M-file Project: HyEQ Toolbox @  Hybrid Systems Laboratory (HSL), 
% https://hybrid.soe.ucsc.edu/software
% http://hybridsimulator.wordpress.com/
%--------------------------------------------------------------------------
% Project: Simulation of a hybrid system
% Description: Jump map
%--------------------------------------------------------------------------
%--------------------------------------------------------------------------
%   See also HYEQSOLVER, PLOTARC, PLOTARC3, PLOTFLOWS, PLOTHARC,
%   PLOTHARCCOLOR, PLOTHARCCOLOR3D, PLOTHYBRIDARC, PLOTJUMPS.
%   Copyright @ Hybrid Systems Laboratory (HSL),
%   Revision: 0.0.0.3 Date: 05/20/2015 3:42:00
%--------------------------------------------------------------------------

xplus = [x(1:13); 1-x(14)];

== matlab function sim_switc_hover_vol_rotation/HSu/jump set D ==
  data: x input; v output; Vi input; a parameter; b parameter
function v  = D(x, Vi, a, b) 
%--------------------------------------------------------------------------
% Matlab M-file Project: HyEQ Toolbox @  Hybrid Systems Laboratory (HSL), 
% https://hybrid.soe.ucsc.edu/software
% http://hybridsimulator.wordpress.com/
%--------------------------------------------------------------------------
% Project: Simulation of a hybrid system
% Description: Jump set
%--------------------------------------------------------------------------
%--------------------------------------------------------------------------
%   See also HYEQSOLVER, PLOTARC, PLOTARC3, PLOTFLOWS, PLOTHARC,
%   PLOTHARCCOLOR, PLOTHARCCOLOR3D, PLOTHYBRIDARC, PLOTJUMPS.
%   Copyright @ Hybrid Systems Laboratory (HSL),
%   Revision: 0.0.0.3 Date: 05/20/2015 3:42:00
%
%state
s = x(14);

if ( ((Vi >= b ) && (s == 0)) || ((Vi <= a ) && (s == 1)))  % jump condition
    v = 1;  % report jump
else
    v = 0;   % do not report jump
end

== matlab function sim_switc_hover_vol_rotation/Controlleur_hover_NL_rot/translational mis ==
  data: f input; f_r input; f_delta output; q_d input; controlleur parameter
function f_delta = trans_mis(f, f_r,  q_d, controlleur)
%#codegen

f_delta = q2dcm(q_d) * controlleur.d_etoile * f - f_r;

== matlab function sim_switc_hover_vol_rotation/Controlleur_hover_L/dem ==
  data: x input; x_ output
function x_ = demux(x)

x_ = x(1:13);

== matlab function sim_switc_hover_vol_rotation/Controlleur_hover_L/Satutation des commandes/convert ==
  data: u input; w1 output; drone parameter; w2 output; d1 output; d2 output
function [w1, w2, d1, d2] = convert(u, drone)
%#codegen
kf = drone.PROP_KP;

T1 = max(u(1),0);
T2 = max(u(2),0);
d1_T1 = u(3);
d2_T2 = u(4);

w1 = sqrt(T1/kf);
w2 = sqrt(T2/kf);
d1 = d1_T1/T1;
d2 = d2_T2/T2;

== matlab function sim_switc_hover_vol_rotation/Controlleur_hover_L/Satutation des commandes/convert1 ==
  data: w1 input; w2 input; d1 input; d2 input; T1_sat output; T2_sat output; drone parameter; d1_t1_sat output; d2_t2_sat output
function [T1_sat, T2_sat, d1_t1_sat, d2_t2_sat] = convert2(w1, w2, d1, d2, drone)
%#codegen
kf = drone.PROP_KP;

T1_sat = kf*w1^2;
d1_t1_sat = d1*T1_sat;
T2_sat = kf*w2^2;
d2_t2_sat = d2*T2_sat;

== matlab function sim_switc_hover_vol_rotation/HSu/Subsystem/MATLAB Function ==
  data: t input; y output
function y = disturbance(t)
    if(t>10)

%         y = [50; zeros(13,1)];
        y = zeros(14,1);
    else
        y = zeros(14,1);
    end
end

== matlab function sim_switc_hover_vol_rotation/Generateur de trajectoire ==
  data: time input; position_cible output; list_point parameter
function position_cible = traj(time, list_point)
%#codegen

position_cible = 1;

== matlab function sim_switc_hover_vol_rotation/Controlleur_vol_NL/MATLAB Function1 ==
  data: u input; y output
function y = fcn(u)
%#codegen

y = norm(u);

== matlab function sim_switc_hover_vol_rotation/Controlleur_vol_NL/Orientation ==
  data: tau output; u_p output; v_norm output; x input; controlleur parameter; drone parameter; u_e output; c_theta output; q_e output; p_cible input
function [tau, u_p, v_norm, u_e, c_theta, q_e]= orientation(x, controlleur, drone, p_cible)
%#codegen
p = x(1:3);
v = x(4:6);
% q  = x(7:10);
wb = x(11:13);

J = drone.INERTIA;


u_p = (p_cible-p)/norm(p_cible-p);
v_norm = v/norm(v);



c_theta = u_p'*v_norm;      %cos (theta)
theta = acos(c_theta);
u_e = cross(u_p, v_norm); 


% q_e = [c_theta; u_e];

q_e = [cos(theta/2);(u_e / norm(u_e))*sin(theta/2)];

% q_e = [sqrt((1+c_theta)/2); (u_e / norm(u_e))*sqrt((1-c_theta)/2)];


tau = -controlleur.kc*sign(q_e(1))*q_e(2:4) + cross(wb, J*wb);
% tau = -controlleur.kc*q_e(1)*q_e(2:4) + cross(wb, J*wb);

== matlab function sim_switc_hover_vol_rotation/state1 ==
  data: x input; p output; v output; q output; wb output; s output
function [p, v,q, wb, s] = demux(x)
%#codegen

p = x(1:3);
v = x(4:6);
q  = x(7:10);
wb = x(11:13);
s = x(14);

== matlab function sim_switc_hover_vol_rotation/Controlleur_vol_NL/Satutation des commandes/convert ==
  data: u input size=4; w1 output; drone parameter; w2 output; d1 output; d2 output
function [w1, w2, d1, d2] = convert(u, drone)
%#codegen
kf = drone.PROP_KP;

T1 = max(u(1),0);
T2 = max(u(2),0);
d1 = u(3);
d2 = u(4);

w1 = sqrt(T1/kf);
w2 = sqrt(T2/kf);

== matlab function sim_switc_hover_vol_rotation/Controlleur_vol_NL/Satutation des commandes/convert1 ==
  data: w1 input; w2 input; d1 input; d2 input; T1_sat output; T2_sat output; drone parameter; d1_sat output; d2_sat output
function [T1_sat, T2_sat, d1_sat, d2_sat] = convert2(w1, w2, d1, d2, drone)
%#codegen
kf = drone.PROP_KP;

T1_sat = kf*w1^2;
d1_sat = d1;
T2_sat = kf*w2^2;
d2_sat = d2;

== matlab function sim_switc_hover_vol_rotation/Controlleur_vol_NL/Select ==
  data: x input; vbx output
function vbx = select(x)
v = x(4:6);
q  = x(7:10);
D = q2dcm(q);

vb = D'*v;
vbx = vb(1);

== matlab function sim_switc_hover_vol_rotation/Controlleur_vol_NL/Speed control ==
  data: speed input; x input; T1pT2 output; controlleur parameter; drone parameter; vb output; G_b output
function [T1pT2, vb, G_b]   = speed_control(speed, x, controlleur, drone)
%#codegen 

% gravity
g = drone.G;
% vehicle mass
m = drone.MASS;
rho = drone.RHO;
% ws = drone.WINGSPAN;
% chord = drone.CHORD;
Swet = drone.WET_SURFACE;
Sdry = drone.DRY_SURFACE;
S = Swet + Sdry;

PHI_fv = drone.PHI(1:3,1:3);


% p = x(1:3);
v = x(4:6);
q  = x(7:10);
w = x(11:13);

eta = sqrt(norm(v)^2);
D = q2dcm(q);

vb = D'*v;
vbx = vb(1);
% vby = vb(2);
% vbz = vb(3);

G_b = D'*[0;0;g];

ay = drone.P_A2_CG(2);
py = drone.P_P2_CG(2);
die_c = drone.PHI(3,3);
Cd0 = drone.PHI(1,1);

Swet   = drone.WET_SURFACE;
Sdry   = drone.DRY_SURFACE;
Sp = pi*drone.PROP_RADIUS^2;
Thetam = drone.ELEVON_MEFFICIENCY(2);
% Thetaf = drone.ELEVON_FEFFICIENCY(2);
kf = drone.PROP_KP;
km = drone.PROP_KM;
S = Swet + Sdry;
rho    = drone.RHO;
phi_n  = drone.PHI_n;
chord  = drone.CHORD;
ws     = drone.WINGSPAN;
B = diag([ws; chord; ws]);
dR = drone.CENTRAGE ;
eta = sqrt( norm(v)^2 + phi_n*norm(B*w)^2 );

% T1pT2 = 1/(2*(1-(Swet/(4*Sp))*Cd0))*rho*S*eta*Cd0*vbx + G_b(1) + controlleur.kv * (speed - vb(1));
 T1pT2 = controlleur.kv * (speed - vb(1));

== matlab function sim_switc_hover_vol_rotation/Controlleur_hover_NL_rot/distri ==
  data: f input; u output; tau_r input; controlleur parameter
function u = dist(f,tau_r, controlleur)
%#codegen
u = controlleur.M_k * tau_r + controlleur.u_barre * f;
